simulink model "PMSM_ClosedLoop_s32k144"  (Simulink 9.0)
settings: Solver=FixedStepDiscrete  StartTime=0.0  StopTime=10  RelTol=1e-3  EnableMultiTasking=on
InitFcn:
  | mbd_s32k_consistency_checks(bdroot(gcs));
undefined symbols (not defined in the file): External, LQFP, One, Shot, TRGMUX_PDB_TRIG
libraries: mbd_s32k1xx_ec_toolbox x50, ammclib_bam_s32k14x x26, simulink x18, mbd_msd_ec_toolbox x5
(part 2 of 2)

== system PMSM_ClosedLoop_s32k144/S32K144 EVB/SlowLoopControl/Compute_Positioning_Mode ==
  Speed_Ref : Inport
  ABS : ammclib_bam_s32k14x/MLIB/bam_flt/MLIB_Abs_FLT
  Data Store Write : DataStoreWrite  DataStoreName=MODE
  Data Store Write2 : DataStoreWrite  DataStoreName=SPEED_REF
  Positioning_Mode : Stateflow chart  TreatAsAtomicUnit=on
      settings: RTWSystemCode=Nonreusable function  RTWFcnNameOpts=Use subsystem name  RTWFileNameOpts=Use subsystem name
  wires:
  Speed_Ref/1 -> ABS/1, Data Store Write2/1
  Positioning_Mode/1(Mode) -> Data Store Write/1
  ABS/1 -> Positioning_Mode/1(SPEED_REF)

== system PMSM_ClosedLoop_s32k144/S32K144 EVB/SlowLoopControl/Generate_Speed_Reference ==
  Speed_Cmd : Inport
  Align Sequence : Stateflow chart  TreatAsAtomicUnit=on
  AlignTimer : DataStoreMemory  DataStoreName=AlignTimer  ReadBeforeWriteMsg=warning  WriteAfterWriteMsg=warning  WriteAfterReadMsg=warning  ShowAdditionalParam=off  OutDataTypeStr=uint16
      settings: RTWStateStorageClass=ExportedGlobal
  AlignTimerIn : DataStoreRead  DataStoreName=AlignTimer
  AlignTimerOut : DataStoreWrite  DataStoreName=AlignTimer
  ExecureAlign : DataStoreWrite  DataStoreName=ExecuteAlign
  GFLIB_Ramp_FLT : ammclib_bam_s32k14x/GFLIB/bam_flt/GFLIB_Ramp_FLT  fltRampUp=0.1  fltRampDown=0.1
  Speed_Ref : Outport
  wires:
  Align Sequence/1(DelayTimeOut) -> AlignTimerOut/1
  AlignTimerIn/1 -> Align Sequence/1(DelayTimeIn)
  Align Sequence/3(ExecuteAlign) -> ExecureAlign/1
  Align Sequence/2(SpeedOut) -> GFLIB_Ramp_FLT/1
  GFLIB_Ramp_FLT/1 -> Speed_Ref/1
  Speed_Cmd/1 -> Align Sequence/2(SpeedIn)

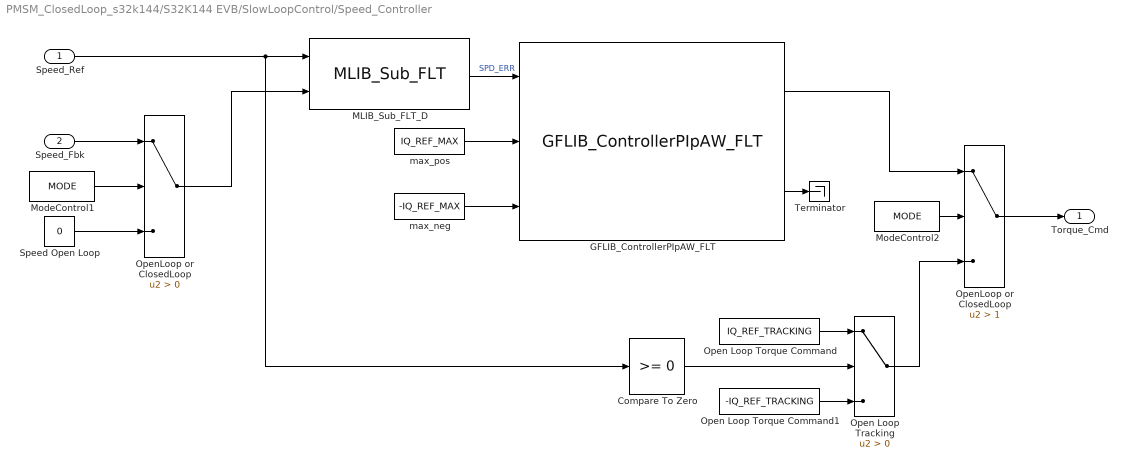
== system PMSM_ClosedLoop_s32k144/S32K144 EVB/SlowLoopControl/Speed_Controller ==
  Speed_Ref : Inport
  Speed_Fbk : Inport  Port=2
  Compare To Zero : simulink/Logic and Bit Operations/Compare To Zero  relop=>=  OutDataTypeStr=boolean
  GFLIB_ControllerPIpAW_FLT : ammclib_bam_s32k14x/GFLIB/bam_flt/GFLIB_ControllerPIpAW_FLT  fltPropGain=0.014207315561740161  fltIntegGain=0.00002231679909799742
  MLIB_Sub_FLT_D : ammclib_bam_s32k14x/MLIB/bam_flt/MLIB_Sub_FLT
  ModeControl1 : DataStoreRead  DataStoreName=MODE
  ModeControl2 : DataStoreRead  DataStoreName=MODE
  Open Loop Torque Command : Constant  Value=IQ_REF_TRACKING  OutDataTypeStr=Inherit: Inherit via back propagation
  Open Loop Torque Command1 : Constant  Value=-IQ_REF_TRACKING  OutDataTypeStr=Inherit: Inherit via back propagation
  Open Loop Tracking : Switch  Criteria=u2 > Threshold
  OpenLoop or ClosedLoop : Switch  Criteria=u2 > Threshold
  "OpenLoop or ClosedLoop " : Switch  Criteria=u2 > Threshold  Threshold=1
  Speed Open Loop : Constant  Value=0  OutDataTypeStr=Inherit: Inherit via back propagation
  Terminator : Terminator
  max_neg : Constant  Value=-IQ_REF_MAX  OutDataTypeStr=Inherit: Inherit via back propagation
  max_pos : Constant  Value=IQ_REF_MAX  OutDataTypeStr=Inherit: Inherit via back propagation
  Torque_Cmd : Outport
  wires:
  Speed_Ref/1 -> MLIB_Sub_FLT_D/1, Compare To Zero/1
  "OpenLoop or ClosedLoop "/1 -> Torque_Cmd/1
  Open Loop Tracking/1 -> "OpenLoop or ClosedLoop "/3
  Open Loop Torque Command/1 -> Open Loop Tracking/1
  Compare To Zero/1 -> Open Loop Tracking/2
  Open Loop Torque Command1/1 -> Open Loop Tracking/3
  GFLIB_ControllerPIpAW_FLT/1 -> "OpenLoop or ClosedLoop "/1
  ModeControl2/1 -> "OpenLoop or ClosedLoop "/2
  Speed Open Loop/1 -> OpenLoop or ClosedLoop/3
  ModeControl1/1 -> OpenLoop or ClosedLoop/2
  OpenLoop or ClosedLoop/1 -> MLIB_Sub_FLT_D/2
  Speed_Fbk/1 -> OpenLoop or ClosedLoop/1
  MLIB_Sub_FLT_D/1 -> GFLIB_ControllerPIpAW_FLT/1  "SPD_ERR"
  GFLIB_ControllerPIpAW_FLT/2 -> Terminator/1
  max_pos/1 -> GFLIB_ControllerPIpAW_FLT/2
  max_neg/1 -> GFLIB_ControllerPIpAW_FLT/3

== system PMSM_ClosedLoop_s32k144/S32K144 EVB/SlowLoopControl/Update_Theta_Offset ==
  Speed_Ref : Inport
  CW vs CCW : Switch  Criteria=u2 > Threshold
  Compare To Zero : simulink/Logic and Bit Operations/Compare To Zero  relop=>=  OutDataTypeStr=boolean
  Constant1 : Constant  Value=pi/2  OutDataTypeStr=Inherit: Inherit via back propagation
  Constant2 : Constant  Value=3*pi/2  OutDataTypeStr=Inherit: Inherit via back propagation
  Theta_Offset : DataStoreWrite  DataStoreName=THETA_OFFSET
  wires:
  Constant2/1 -> CW vs CCW/3
  CW vs CCW/1 -> Theta_Offset/1
  Compare To Zero/1 -> CW vs CCW/2
  Constant1/1 -> CW vs CCW/1
  Speed_Ref/1 -> Compare To Zero/1

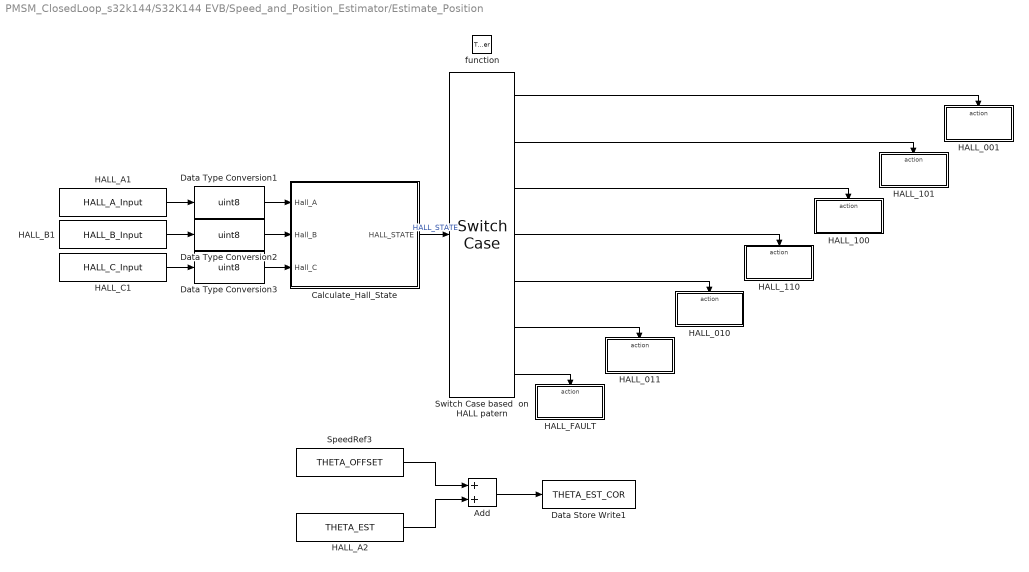
== system PMSM_ClosedLoop_s32k144/S32K144 EVB/Speed_and_Position_Estimator/Estimate_Position ==
  function : TriggerPort  TriggerType=function-call  VariantControl=(inherit)
  Add : Sum
  Calculate_Hall_State : Subsystem  Priority=1
  Data Store Write1 : DataStoreWrite  Priority=20  DataStoreName=THETA_EST_COR
  Data Type Conversion1 : DataTypeConversion  OutDataTypeStr=uint8
  Data Type Conversion2 : DataTypeConversion  OutDataTypeStr=uint8
  Data Type Conversion3 : DataTypeConversion  OutDataTypeStr=uint8
  HALL_001 : Subsystem  TreatAsAtomicUnit=on
  HALL_010 : Subsystem  TreatAsAtomicUnit=on
  HALL_011 : Subsystem  TreatAsAtomicUnit=on
  HALL_100 : Subsystem  TreatAsAtomicUnit=on
  HALL_101 : Subsystem  TreatAsAtomicUnit=on
  HALL_110 : Subsystem  TreatAsAtomicUnit=on
  HALL_A1 : DataStoreRead  DataStoreName=HALL_A_Input
  HALL_A2 : DataStoreRead  DataStoreName=THETA_EST
  HALL_B1 : DataStoreRead  DataStoreName=HALL_B_Input
  HALL_C1 : DataStoreRead  DataStoreName=HALL_C_Input
  HALL_FAULT : Subsystem  TreatAsAtomicUnit=on
  SpeedRef3 : DataStoreRead  DataStoreName=THETA_OFFSET
  Switch Case based  on HALL patern : SwitchCase  Priority=2  CaseConditions={1, 5, 4, 6, 2, 3}
  wires:
  Data Type Conversion2/1 -> Calculate_Hall_State/2(Hall_B)
  HALL_A1/1 -> Data Type Conversion1/1
  HALL_C1/1 -> Data Type Conversion3/1
  Data Type Conversion3/1 -> Calculate_Hall_State/3(Hall_C)
  Data Type Conversion1/1 -> Calculate_Hall_State/1(Hall_A)
  HALL_B1/1 -> Data Type Conversion2/1
  Calculate_Hall_State/1(HALL_STATE) -> Switch Case based  on HALL patern/1  "HALL_STATE"
  Switch Case based  on HALL patern/1 -> HALL_001/Action
  Switch Case based  on HALL patern/2 -> HALL_101/Action
  Switch Case based  on HALL patern/3 -> HALL_100/Action
  Switch Case based  on HALL patern/4 -> HALL_110/Action
  Switch Case based  on HALL patern/5 -> HALL_010/Action
  Switch Case based  on HALL patern/6 -> HALL_011/Action
  SpeedRef3/1 -> Add/1
  HALL_A2/1 -> Add/2
  Add/1 -> Data Store Write1/1
  Switch Case based  on HALL patern/7 -> HALL_FAULT/Action

== system PMSM_ClosedLoop_s32k144/S32K144 EVB/Speed_and_Position_Estimator/Update_HALL_A ==
  function : TriggerPort  TriggerType=function-call  VariantControl=(inherit)
  Data Store Read1 : DataStoreRead  DataStoreName=HALL_A_Input
  Data Store Write1 : DataStoreWrite  DataStoreName=HALL_A_Input
  Function-Call Generator : simulink/Ports & Subsystems/Function-Call Generator  sample_time=-1  numberOfIterations=1
  Logical Operator : Logic  Operator=NOT  AllPortsSameDT=off  OutDataTypeStr=boolean
  Call : Outport
  wires:
  Function-Call Generator/1 -> Call/1
  Data Store Read1/1 -> Logical Operator/1
  Logical Operator/1 -> Data Store Write1/1

== system PMSM_ClosedLoop_s32k144/S32K144 EVB/Speed_and_Position_Estimator/Update_HALL_B ==
  function : TriggerPort  TriggerType=function-call  VariantControl=(inherit)
  Data Store Read1 : DataStoreRead  DataStoreName=HALL_B_Input
  Data Store Write1 : DataStoreWrite  DataStoreName=HALL_B_Input
  Function-Call Generator : simulink/Ports & Subsystems/Function-Call Generator  sample_time=-1  numberOfIterations=1
  Logical Operator : Logic  Operator=NOT  AllPortsSameDT=off  OutDataTypeStr=boolean
  Call : Outport
  wires:
  Logical Operator/1 -> Data Store Write1/1
  Data Store Read1/1 -> Logical Operator/1
  Function-Call Generator/1 -> Call/1

== system PMSM_ClosedLoop_s32k144/S32K144 EVB/Speed_and_Position_Estimator/Update_HALL_C_Estimate_Speed ==
  function : TriggerPort  TriggerType=function-call  VariantControl=(inherit)
  Compute_Estimated_Speed : Subsystem  TreatAsAtomicUnit=on
  Data Store Read1 : DataStoreRead  Priority=0  DataStoreName=HALL_C_Input
  Data Store Write1 : DataStoreWrite  DataStoreName=HALL_C_Input
  Function-Call Generator : simulink/Ports & Subsystems/Function-Call Generator  sample_time=-1  numberOfIterations=1
  If : If  Priority=1  IfExpression=u1 == 1  ShowElse=off
  Logical Operator : Logic  Priority=2  Operator=NOT  AllPortsSameDT=off  OutDataTypeStr=boolean
  Call : Outport
  Speed_Fbk : Outport  Port=2
  wires:
  Function-Call Generator/1 -> Call/1
  Data Store Read1/1 -> If/1, Logical Operator/1
  Logical Operator/1 -> Data Store Write1/1
  If/1 -> Compute_Estimated_Speed/Action
  Compute_Estimated_Speed/1(Speed_Fbk) -> Speed_Fbk/1

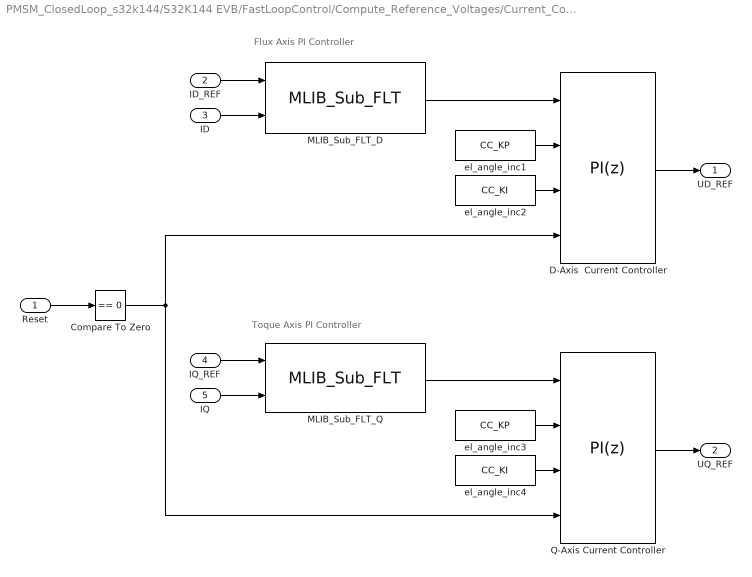
== system PMSM_ClosedLoop_s32k144/S32K144 EVB/FastLoopControl/Compute_Reference_Voltages/Current_Controllers_DQ ==
  note: Flux Axis PI Controller
  note: Toque Axis PI Controller
  Reset : Inport
  ID_REF : Inport  Port=2
  ID : Inport  Port=3
  IQ_REF : Inport  Port=4
  IQ : Inport  Port=5
  " D-Axis  Current Controller" : simulink/Continuous/PID Controller  Controller=PI  Form=Parallel  TimeDomain=Discrete-time  SampleTime=-1  IntegratorMethod=Forward Euler  FilterMethod=Forward Euler  ControllerParametersSource=external  P=1  I=1  D=0  UseFilter=on  N=100  TunerSelectOption=Transfer Function Based (PID Tuner App)  ZeroCross=off  InitialConditionSource=internal  InitialConditionForIntegrator=0  InitialConditionForFilter=0  DifferentiatorICPrevScaledInput=0  ExternalReset=rising  TrackingMode=off  Kt=1  LimitOutput=on  UpperSaturationLimit=0.9  LowerSaturationLimit=-0.9  LinearizeAsGain=off  AntiWindupMode=none  Kb=1  RndMeth=Simplest  POutMin=[]  POutMax=[]  IOutMin=[]  IOutMax=[]  DOutMin=[]  DOutMax=[]  NOutMin=[]  NOutMax=[]  SumOutMin=[]  SumOutMax=[]  SaturationOutMin=[]  SaturationOutMax=[]  PParamMin=[]  PParamMax=[]  IParamMin=[]  IParamMax=[]  DParamMin=[]  DParamMax=[]  NParamMin=[]  NParamMax=[]  KbParamMin=[]  KbParamMax=[]  KtParamMin=[]  KtParamMax=[]  KbOutMin=[]  KbOutMax=[]  KtOutMin=[]  KtOutMax=[]  IntegratorOutMin=[]  IntegratorOutMax=[]  FilterOutMin=[]  FilterOutMax=[]  SumI1OutMin=[]  SumI1OutMax=[]  SumI2OutMin=[]  SumI2OutMax=[]  SumI3OutMin=[]  SumI3OutMax=[]  SumDOutMin=[]  SumDOutMax=[]  DifferentiatorOutMin=[]  DifferentiatorOutMax=[]  FilterDiffOutCoefMin=[]  FilterDiffOutCoefMax=[]  ReciprocalOutMin=[]  ReciprocalOutMax=[]  SumDenOutMin=[]  SumDenOutMax=[]  SumNumOutMin=[]  SumNumOutMax=[]  DivideOutMin=[]  DivideOutMax=[]  IntegratorContinuousStateAttributes=''  IntegratorStateMustResolveToSignalObject=off  IntegratorRTWStateStorageClass=Auto  FilterContinuousStateAttributes=''  FilterStateMustResolveToSignalObject=off  FilterRTWStateStorageClass=Auto
  Compare To Zero : simulink/Logic and Bit Operations/Compare To Zero  relop===  OutDataTypeStr=boolean
  MLIB_Sub_FLT_D : ammclib_bam_s32k14x/MLIB/bam_flt/MLIB_Sub_FLT
  MLIB_Sub_FLT_Q : ammclib_bam_s32k14x/MLIB/bam_flt/MLIB_Sub_FLT
  Q-Axis Current Controller : simulink/Continuous/PID Controller  Controller=PI  Form=Parallel  TimeDomain=Discrete-time  SampleTime=-1  IntegratorMethod=Forward Euler  FilterMethod=Forward Euler  ControllerParametersSource=external  P=1  I=1  D=0  UseFilter=on  N=100  TunerSelectOption=Transfer Function Based (PID Tuner App)  ZeroCross=off  InitialConditionSource=internal  InitialConditionForIntegrator=0  InitialConditionForFilter=0  DifferentiatorICPrevScaledInput=0  ExternalReset=rising  TrackingMode=off  Kt=1  LimitOutput=on  UpperSaturationLimit=0.9  LowerSaturationLimit=-0.9  LinearizeAsGain=off  AntiWindupMode=clamping  Kb=1  RndMeth=Simplest  POutMin=[]  POutMax=[]  IOutMin=[]  IOutMax=[]  DOutMin=[]  DOutMax=[]  NOutMin=[]  NOutMax=[]  SumOutMin=[]  SumOutMax=[]  SaturationOutMin=[]  SaturationOutMax=[]  PParamMin=[]  PParamMax=[]  IParamMin=[]  IParamMax=[]  DParamMin=[]  DParamMax=[]  NParamMin=[]  NParamMax=[]  KbParamMin=[]  KbParamMax=[]  KtParamMin=[]  KtParamMax=[]  KbOutMin=[]  KbOutMax=[]  KtOutMin=[]  KtOutMax=[]  IntegratorOutMin=[]  IntegratorOutMax=[]  FilterOutMin=[]  FilterOutMax=[]  SumI1OutMin=[]  SumI1OutMax=[]  SumI2OutMin=[]  SumI2OutMax=[]  SumI3OutMin=[]  SumI3OutMax=[]  SumDOutMin=[]  SumDOutMax=[]  DifferentiatorOutMin=[]  DifferentiatorOutMax=[]  FilterDiffOutCoefMin=[]  FilterDiffOutCoefMax=[]  ReciprocalOutMin=[]  ReciprocalOutMax=[]  SumDenOutMin=[]  SumDenOutMax=[]  SumNumOutMin=[]  SumNumOutMax=[]  DivideOutMin=[]  DivideOutMax=[]  IntegratorContinuousStateAttributes=''  IntegratorStateMustResolveToSignalObject=off  IntegratorRTWStateStorageClass=Auto  FilterContinuousStateAttributes=''  FilterStateMustResolveToSignalObject=off  FilterRTWStateStorageClass=Auto
  el_angle_inc1 : DataStoreRead  DataStoreName=CC_KP
  el_angle_inc2 : DataStoreRead  DataStoreName=CC_KI
  el_angle_inc3 : DataStoreRead  DataStoreName=CC_KP
  el_angle_inc4 : DataStoreRead  DataStoreName=CC_KI
  UD_REF : Outport
  UQ_REF : Outport  Port=2
  wires:
  MLIB_Sub_FLT_D/1 -> " D-Axis  Current Controller"/1
  el_angle_inc1/1 -> " D-Axis  Current Controller"/2
  el_angle_inc2/1 -> " D-Axis  Current Controller"/3
  ID_REF/1 -> MLIB_Sub_FLT_D/1
  MLIB_Sub_FLT_Q/1 -> Q-Axis Current Controller/1
  el_angle_inc3/1 -> Q-Axis Current Controller/2
  el_angle_inc4/1 -> Q-Axis Current Controller/3
  ID/1 -> MLIB_Sub_FLT_D/2
  IQ_REF/1 -> MLIB_Sub_FLT_Q/1
  IQ/1 -> MLIB_Sub_FLT_Q/2
  " D-Axis  Current Controller"/1 -> UD_REF/1
  Q-Axis Current Controller/1 -> UQ_REF/1
  Reset/1 -> Compare To Zero/1
  Compare To Zero/1 -> Q-Axis Current Controller/4, " D-Axis  Current Controller"/4

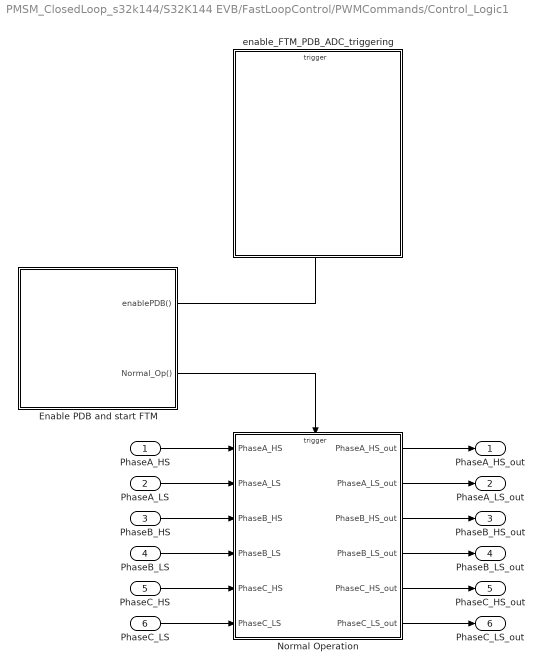
== system PMSM_ClosedLoop_s32k144/S32K144 EVB/FastLoopControl/PWMCommands/Control_Logic1 ==
  PhaseA_HS : Inport
  PhaseA_LS : Inport  Port=2
  PhaseB_HS : Inport  Port=3
  PhaseB_LS : Inport  Port=4
  PhaseC_HS : Inport  Port=5
  PhaseC_LS : Inport  Port=6
  Enable PDB and start FTM : Stateflow chart  TreatAsAtomicUnit=on
  Normal Operation : Subsystem  TreatAsAtomicUnit=on
  enable_FTM_PDB_ADC_triggering : Subsystem  TreatAsAtomicUnit=on
      settings: RTWSystemCode=Inline
  PhaseA_HS_out : Outport
  PhaseA_LS_out : Outport  Port=2
  PhaseB_HS_out : Outport  Port=3
  PhaseB_LS_out : Outport  Port=4
  PhaseC_HS_out : Outport  Port=5
  PhaseC_LS_out : Outport  Port=6
  wires:
  Enable PDB and start FTM/2(Normal_Op()) -> Normal Operation/Trigger
  Enable PDB and start FTM/1(enablePDB()) -> enable_FTM_PDB_ADC_triggering/Trigger
  PhaseB_HS/1 -> Normal Operation/3(PhaseB_HS)
  PhaseB_LS/1 -> Normal Operation/4(PhaseB_LS)
  PhaseA_LS/1 -> Normal Operation/2(PhaseA_LS)
  PhaseC_HS/1 -> Normal Operation/5(PhaseC_HS)
  PhaseA_HS/1 -> Normal Operation/1(PhaseA_HS)
  PhaseC_LS/1 -> Normal Operation/6(PhaseC_LS)
  Normal Operation/6(PhaseC_LS_out) -> PhaseC_LS_out/1
  Normal Operation/5(PhaseC_HS_out) -> PhaseC_HS_out/1
  Normal Operation/4(PhaseB_LS_out) -> PhaseB_LS_out/1
  Normal Operation/3(PhaseB_HS_out) -> PhaseB_HS_out/1
  Normal Operation/2(PhaseA_LS_out) -> PhaseA_LS_out/1
  Normal Operation/1(PhaseA_HS_out) -> PhaseA_HS_out/1

== system PMSM_ClosedLoop_s32k144/S32K144 EVB/FastLoopControl/Rotor_Position/ComputeElectricAngle ==
  Speed_Reference [rad/s] : Inport
  DIV : ammclib_bam_s32k14x/MLIB/bam_flt/MLIB_Div_FLT
  GFLIB_IntegratorTR_F32 : ammclib_bam_s32k14x/GFLIB/bam_f32/GFLIB_IntegratorTR_F32  f32C1=(2*pi/60)*PP*Nmax*(C_LST/2/pi)*(2^31)  u16NShift=0
  MLIB_ConvertPU_F32FLT : ammclib_bam_s32k14x/MLIB/bam_f32/MLIB_ConvertPU_F32FLT
  MLIB_ConvertPU_FLTF32 : ammclib_bam_s32k14x/MLIB/bam_flt/MLIB_ConvertPU_FLTF32
  MUL : ammclib_bam_s32k14x/MLIB/bam_flt/MLIB_Mul_FLT
  SpeedMax_rad/s : Constant  Value=Nmax*(2*pi/60)  OutDataTypeStr=Inherit: Inherit via back propagation
  pi : Constant  Value=pi  OutDataTypeStr=Inherit: Inherit via back propagation
  theta : Outport  OutDataTypeStr=single
  wires:
  pi/1 -> MUL/2
  GFLIB_IntegratorTR_F32/1 -> MLIB_ConvertPU_FLTF32/1
  MLIB_ConvertPU_F32FLT/1 -> GFLIB_IntegratorTR_F32/1
  MLIB_ConvertPU_FLTF32/1 -> MUL/1
  MUL/1 -> theta/1
  Speed_Reference [rad/s]/1 -> DIV/1
  DIV/1 -> MLIB_ConvertPU_F32FLT/1
  SpeedMax_rad/s/1 -> DIV/2

== system PMSM_ClosedLoop_s32k144/S32K144 EVB/IO Controls/NormalOp/FAULT ==
  Action Port : ActionPort
  LED_BLUE : mbd_s32k1xx_ec_toolbox/GPIO Blocks/Digital_Output  gpio_pin=PTD0: [PTD0 | Port D I/O]  init_val=Low  drive_strength=Low
  LED_RED : mbd_s32k1xx_ec_toolbox/GPIO Blocks/Digital_Output  gpio_pin=PTD15: [PTD15 | Port D I/O]  init_val=Low  drive_strength=Low
  OFF : Constant  OutDataTypeStr=boolean
  ON : Constant  Value=0  OutDataTypeStr=boolean
  wires:
  OFF/1 -> LED_BLUE/1
  ON/1 -> LED_RED/1

== system PMSM_ClosedLoop_s32k144/S32K144 EVB/IO Controls/NormalOp/RUNNING_OK ==
  Action Port : ActionPort
  LED_BLUE : mbd_s32k1xx_ec_toolbox/GPIO Blocks/Digital_Output  gpio_pin=PTD0: [PTD0 | Port D I/O]  init_val=Low  drive_strength=Low
  LED_RED : mbd_s32k1xx_ec_toolbox/GPIO Blocks/Digital_Output  gpio_pin=PTD15: [PTD15 | Port D I/O]  init_val=Low  drive_strength=Low
  OFF : Constant  OutDataTypeStr=boolean
  ON : Constant  Value=0  OutDataTypeStr=boolean
  wires:
  OFF/1 -> LED_RED/1
  ON/1 -> LED_BLUE/1

== system PMSM_ClosedLoop_s32k144/S32K144 EVB/IO Controls/WaitForStart/Check_Hall_Error ==
  H1 : Inport
  H2 : Inport  Port=2
  H3 : Inport  Port=3
  Add : Sum  Inputs=+++
  Compare To Constant : simulink/Logic and Bit Operations/Compare To Constant  relop===  const=3  OutDataTypeStr=boolean
  Compare To Constant1 : simulink/Logic and Bit Operations/Compare To Constant  relop===  const=0  OutDataTypeStr=boolean
  Logical Operator : Logic  Operator=OR  AllPortsSameDT=off  OutDataTypeStr=boolean
  Hall_Errorr : Outport
  wires:
  Logical Operator/1 -> Hall_Errorr/1
  Compare To Constant1/1 -> Logical Operator/2
  H3/1 -> Add/3
  Add/1 -> Compare To Constant1/1, Compare To Constant/1
  H2/1 -> Add/2
  Compare To Constant/1 -> Logical Operator/1
  H1/1 -> Add/1

== system PMSM_ClosedLoop_s32k144/S32K144 EVB/IO Controls/WaitForStart/HALL_FAULT ==
  Action Port : ActionPort
  Data Store Write2 : DataStoreWrite  DataStoreName=HALL_ERROR
  "NOK " : Constant  OutDataTypeStr=uint8
  wires:
  "NOK "/1 -> Data Store Write2/1

== system PMSM_ClosedLoop_s32k144/S32K144 EVB/IRQ_Dispatcher/Generate_Triggers/Keep_Counting ==
  LoopCounter : Inport
  Action Port : ActionPort
  LoopCounter_save : DataStoreWrite  DataStoreName=LoopCounter
  wires:
  LoopCounter/1 -> LoopCounter_save/1

== system PMSM_ClosedLoop_s32k144/S32K144 EVB/IRQ_Dispatcher/Generate_Triggers/Trigger_SlowLoop_Execution ==
  Action Port : ActionPort
  Function-Call Generator : simulink/Ports & Subsystems/Function-Call Generator  sample_time=-1  numberOfIterations=1
  LoopCounter_reset : DataStoreWrite  DataStoreName=LoopCounter
  reset_to_zero : Constant  Value=0  OutDataTypeStr=uint16
  Call : Outport
  wires:
  Function-Call Generator/1 -> Call/1
  reset_to_zero/1 -> LoopCounter_reset/1

== system PMSM_ClosedLoop_s32k144/S32K144 EVB/Measurements/FaultDetection/FAILURE ==
  Action Port : ActionPort
  Compare To Two : simulink/Logic and Bit Operations/Compare To Constant  relop=>=  const=2  OutDataTypeStr=boolean
  FAULT_read : DataStoreRead  DataStoreName=FAULT
  Failed Subsystem : Subsystem  TreatAsAtomicUnit=on
  If : If  NumInputs=2  IfExpression=(u1 == 1)&(u2==1)  ShowElse=off
  LoopCounter_read : DataStoreRead  DataStoreName=LoopCounter
  wires:
  If/1 -> Failed Subsystem/Action
  LoopCounter_read/1 -> Compare To Two/1
  FAULT_read/1 -> If/1
  Compare To Two/1 -> If/2

== system PMSM_ClosedLoop_s32k144/S32K144 EVB/Speed_and_Position_Estimator/Estimate_Position/Calculate_Hall_State ==
  Hall_A : Inport
  Hall_B : Inport  Port=2
  Hall_C : Inport  Port=3
  Gain1 : Gain  Gain=4  OutDataTypeStr=uint8  ParamDataTypeStr=Inherit: Same as input
  Gain2 : Gain  Gain=2  OutDataTypeStr=uint8  ParamDataTypeStr=Inherit: Same as input
  Sum : Sum  Inputs=+++  AccumDataTypeStr=uint8  OutDataTypeStr=uint8  InputSameDT=on
  HALL_STATE : Outport
  wires:
  Sum/1 -> HALL_STATE/1
  Gain2/1 -> Sum/2
  Gain1/1 -> Sum/1
  Hall_A/1 -> Gain1/1
  Hall_B/1 -> Gain2/1
  Hall_C/1 -> Sum/3

== system PMSM_ClosedLoop_s32k144/S32K144 EVB/Speed_and_Position_Estimator/Estimate_Position/HALL_001 ==
  Action Port : ActionPort
  -180deg : Constant  Value=-pi  OutDataTypeStr=Inherit: Inherit via back propagation
  Data Store Write4 : DataStoreWrite  DataStoreName=THETA_EST
  wires:
  -180deg/1 -> Data Store Write4/1

== system PMSM_ClosedLoop_s32k144/S32K144 EVB/Speed_and_Position_Estimator/Estimate_Position/HALL_010 ==
  Action Port : ActionPort
  60deg : Constant  Value=pi/3  OutDataTypeStr=Inherit: Inherit via back propagation
  Data Store Write4 : DataStoreWrite  DataStoreName=THETA_EST
  wires:
  60deg/1 -> Data Store Write4/1

== system PMSM_ClosedLoop_s32k144/S32K144 EVB/Speed_and_Position_Estimator/Estimate_Position/HALL_011 ==
  Action Port : ActionPort
  120deg : Constant  Value=2*pi/3  OutDataTypeStr=Inherit: Inherit via back propagation
  Data Store Write4 : DataStoreWrite  DataStoreName=THETA_EST
  wires:
  120deg/1 -> Data Store Write4/1

== system PMSM_ClosedLoop_s32k144/S32K144 EVB/Speed_and_Position_Estimator/Estimate_Position/HALL_100 ==
  Action Port : ActionPort
  -60deg : Constant  Value=-pi/3  OutDataTypeStr=Inherit: Inherit via back propagation
  Data Store Write4 : DataStoreWrite  DataStoreName=THETA_EST
  wires:
  -60deg/1 -> Data Store Write4/1

== system PMSM_ClosedLoop_s32k144/S32K144 EVB/Speed_and_Position_Estimator/Estimate_Position/HALL_101 ==
  Action Port : ActionPort
  -120deg : Constant  Value=-2*pi/3  OutDataTypeStr=Inherit: Inherit via back propagation
  Data Store Write4 : DataStoreWrite  DataStoreName=THETA_EST
  wires:
  -120deg/1 -> Data Store Write4/1

== system PMSM_ClosedLoop_s32k144/S32K144 EVB/Speed_and_Position_Estimator/Estimate_Position/HALL_110 ==
  Action Port : ActionPort
  0deg : Constant  Value=0  OutDataTypeStr=Inherit: Inherit via back propagation
  Data Store Write4 : DataStoreWrite  DataStoreName=THETA_EST
  wires:
  0deg/1 -> Data Store Write4/1

== system PMSM_ClosedLoop_s32k144/S32K144 EVB/Speed_and_Position_Estimator/Estimate_Position/HALL_FAULT ==
  Action Port : ActionPort
  Data Store Write1 : DataStoreWrite  DataStoreName=FAULT
  Data Store Write2 : DataStoreWrite  DataStoreName=HALL_ERROR
  FTM_PWM_Disable_Enable : mbd_s32k1xx_ec_toolbox/Motor Control Blocks/FTM Blocks/FTM_PWM_Disable_Enable  ftmModule=3  action=Disable
  NOK : Constant  OutDataTypeStr=boolean
  "NOK " : Constant  OutDataTypeStr=uint8
  wires:
  NOK/1 -> Data Store Write1/1
  "NOK "/1 -> Data Store Write2/1

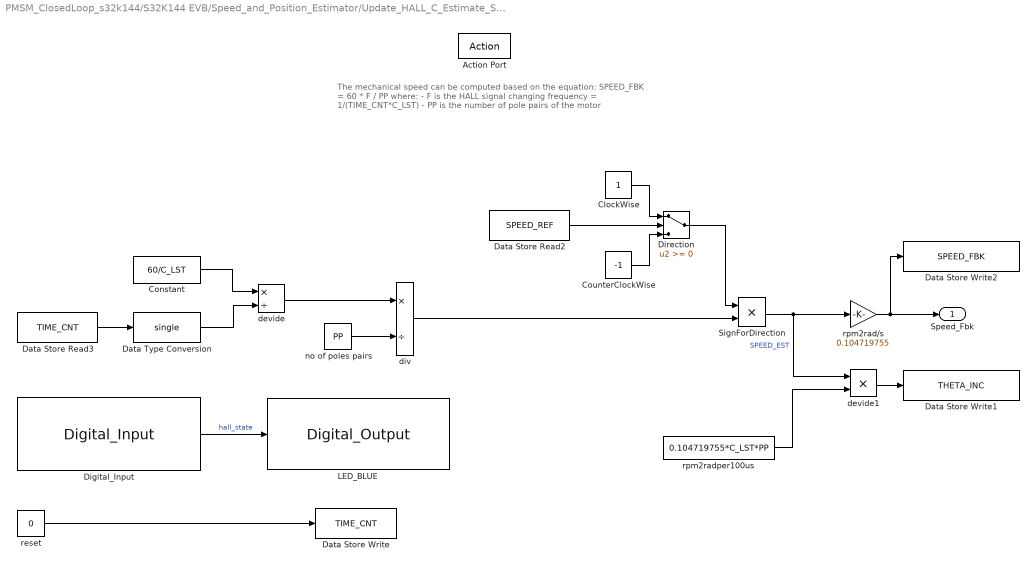
== system PMSM_ClosedLoop_s32k144/S32K144 EVB/Speed_and_Position_Estimator/Update_HALL_C_Estimate_Speed/Compute_Estimated_Speed ==
  note: The mechanical speed can be computed based on the equation:
      | SPEED_FBK = 60 * F / PP
      | where:
      | - F is the HALL signal changing frequency = 1/(TIME_CNT*C_LST)
      | - PP is the number of pole pairs of the motor
  Action Port : ActionPort
  ClockWise : Constant  OutDataTypeStr=Inherit: Inherit via back propagation
  Constant : Constant  Value=60/C_LST  OutDataTypeStr=single
  CounterClockWise : Constant  Value=-1  OutDataTypeStr=Inherit: Inherit via back propagation
  Data Store Read2 : DataStoreRead  DataStoreName=SPEED_REF
  Data Store Read3 : DataStoreRead  DataStoreName=TIME_CNT
  Data Store Write : DataStoreWrite  DataStoreName=TIME_CNT
  Data Store Write1 : DataStoreWrite  Priority=1  DataStoreName=THETA_INC
  Data Store Write2 : DataStoreWrite  Priority=1  DataStoreName=SPEED_FBK
  Data Type Conversion : DataTypeConversion  OutDataTypeStr=single
  Digital_Input : mbd_s32k1xx_ec_toolbox/GPIO Blocks/Digital_Input  gpio_pin=PTA1: [PTA1 | Port A I/O]  pull_resistor=None  passive_filter=off
  Direction : Switch  OutDataTypeStr=single
  LED_BLUE : mbd_s32k1xx_ec_toolbox/GPIO Blocks/Digital_Output  gpio_pin=PTD0: [PTD0 | Port D I/O]  init_val=Low  drive_strength=Low
  SignForDirection : Product  Inputs=**  OutDataTypeStr=single  RndMeth=Zero
  devide : Product  Inputs=*/  OutDataTypeStr=single
  devide1 : Product  Inputs=**  OutDataTypeStr=single
  div : Product  Priority=0  Inputs=*/  OutDataTypeStr=single
  no of poles pairs : Constant  Value=PP  OutDataTypeStr=single
  reset : Constant  Value=0  OutDataTypeStr=uint32
  rpm2rad/s : Gain  Gain=0.104719755
  rpm2radper100us : Constant  Value=0.104719755*C_LST*PP  OutDataTypeStr=single
  Speed_Fbk : Outport
  wires:
  Data Store Read3/1 -> Data Type Conversion/1
  Data Type Conversion/1 -> devide/2
  Constant/1 -> devide/1
  devide/1 -> div/1
  no of poles pairs/1 -> div/2
  Data Store Read2/1 -> Direction/2
  ClockWise/1 -> Direction/1
  CounterClockWise/1 -> Direction/3
  Direction/1 -> SignForDirection/1
  SignForDirection/1 -> rpm2rad/s/1, devide1/1  "SPEED_EST"
  div/1 -> SignForDirection/2
  reset/1 -> Data Store Write/1
  rpm2radper100us/1 -> devide1/2
  devide1/1 -> Data Store Write1/1
  Digital_Input/1 -> LED_BLUE/1  "hall_state"
  rpm2rad/s/1 -> Data Store Write2/1, Speed_Fbk/1

== system PMSM_ClosedLoop_s32k144/S32K144 EVB/FastLoopControl/PWMCommands/Control_Logic1/Normal Operation ==
  PhaseA_HS : Inport
  PhaseA_LS : Inport  Port=2
  PhaseB_HS : Inport  Port=3
  PhaseB_LS : Inport  Port=4
  PhaseC_HS : Inport  Port=5
  PhaseC_LS : Inport  Port=6
  function : TriggerPort  TriggerType=function-call  VariantControl=(inherit)
  PhaseA_HS_out : Outport
  PhaseA_LS_out : Outport  Port=2
  PhaseB_HS_out : Outport  Port=3
  PhaseB_LS_out : Outport  Port=4
  PhaseC_HS_out : Outport  Port=5
  PhaseC_LS_out : Outport  Port=6
  wires:
  PhaseA_HS/1 -> PhaseA_HS_out/1
  PhaseA_LS/1 -> PhaseA_LS_out/1
  PhaseB_HS/1 -> PhaseB_HS_out/1
  PhaseB_LS/1 -> PhaseB_LS_out/1
  PhaseC_HS/1 -> PhaseC_HS_out/1
  PhaseC_LS/1 -> PhaseC_LS_out/1

== system PMSM_ClosedLoop_s32k144/S32K144 EVB/FastLoopControl/PWMCommands/Control_Logic1/enable_FTM_PDB_ADC_triggering ==
  function : TriggerPort  TriggerType=function-call  VariantControl=(inherit)
  Custom code to reload the PDB value : Subsystem  Priority=6  mask(System Outputs){ShowInLibBrowser=0}
      mask prompts: ShowInLibBrowser "Simulink:masks:CustCodeMaskParam1_MP"
      settings: CopyFcn=cccopyfcn(gcb)  OpenFcn=ccopenfcn('System Outputs Function')
      mask Help: eval('feval(''rtwprivate'',''rtwhelpview'',''rtw_sys_outputs_block'')');
      mask Display: disp('System\nOutputs');
  FTM_Init_Trigger_Disable_Enable : mbd_s32k1xx_ec_toolbox/Motor Control Blocks/FTM Blocks/FTM_Init_Trigger_Disable_Enable  Priority=3  ftmModule=3  action=Enable
  FTM_PWM_Disable_Enable : mbd_s32k1xx_ec_toolbox/Motor Control Blocks/FTM Blocks/FTM_PWM_Disable_Enable  Priority=1  ftmModule=3  action=Enable
  ON : Constant  Priority=2  OutDataTypeStr=boolean
  PDB0_Enable : mbd_s32k1xx_ec_toolbox/Motor Control Blocks/PDB Blocks/PDB_Enable  Priority=4  pdbModule=0  pdbAction=Enable
  PDB1_Enable : mbd_s32k1xx_ec_toolbox/Motor Control Blocks/PDB Blocks/PDB_Enable  Priority=5  pdbModule=1  pdbAction=Enable
  "SpeedCmd " : DataStoreWrite  DataStoreName=READY
  TPP_ISR_Enable_Disable 1 : mbd_msd_ec_toolbox/TPP/TPP_ISR_Enable_Disable  Priority=7  tppInstance=0  mcuTppIntEn=on  prioInt=15
  wires:
  ON/1 -> "SpeedCmd "/1

== system PMSM_ClosedLoop_s32k144/S32K144 EVB/Measurements/FaultDetection/FAILURE/Failed Subsystem ==
  Action Port : ActionPort
  FAULT_write : DataStoreWrite  DataStoreName=FAULT
  FTM_PWM_Disable_Enable : mbd_s32k1xx_ec_toolbox/Motor Control Blocks/FTM Blocks/FTM_PWM_Disable_Enable  Priority=1  ftmModule=3  action=Disable
  NOK : Constant  OutDataTypeStr=boolean
  TPP_Functional_Mode : mbd_msd_ec_toolbox/TPP/TPP_Functional_Mode  tppInstance=0  action=Sleep
  wires:
  NOK/1 -> FAULT_write/1

== system PMSM_ClosedLoop_s32k144/S32K144 EVB/FastLoopControl/PWMCommands/Control_Logic1/enable_FTM_PDB_ADC_triggering/Custom code to reload the PDB value ==

== stateflow chart S32K144 EVB/SlowLoopControl/Generate_Speed_Reference/Align Sequence ==
  settings: sampleTime=0.500
  note: Delay for 3 seconds.
  (default) -> (junction 9)
  (junction 9) -> (junction 10) [order 1] : [DelayTimeIn > 3000]
      | {SpeedOut = SpeedIn;
      | ExecuteAlign = 0;}
  (junction 9) -> (junction 11) [order 2]
  (junction 10) -> (junction 12)
  (junction 11) -> (junction 12) : {SpeedOut = 0;
      | DelayTimeOut = DelayTimeIn + 1;
      | ExecuteAlign = 1;}
  data: DelayTimeOut output uint16; DelayTimeIn input uint16; SpeedOut output single; SpeedIn input single; ExecuteAlign output boolean

== stateflow chart S32K144 EVB/FastLoopControl/PWMCommands/Control_Logic1/Enable PDB and start FTM ==
  settings: sampleTime=0.500
  state END
  state A
  (default) -> A
  A -> END : /*Post initializations*/
      | {enablePDB;}
  END -> END : {Normal_Op;}
  events: enablePDB output FUNCTION_CALL_EVENT; Normal_Op output FUNCTION_CALL_EVENT

== stateflow chart S32K144 EVB/SlowLoopControl/Compute_Positioning_Mode/Positioning_Mode ==
  note: Force Mode = 0 when speed is below specified value
      | Tracking Mode = 1 when speed is between specified values
      | Sensor/Sensorless Mode = 2 when speed is above specified value
  (default) -> (junction 34)
  (junction 34) -> (junction 35) [order 1] : [SPEED_REF < FORCE_MODE_SPEED] /* rad/s */
      | {Mode = 0;}
  (junction 34) -> (junction 36) [order 2]
  (junction 35) -> (junction 37)
  (junction 36) -> (junction 37) [order 1] : [(SPEED_REF >= (FORCE_MODE_SPEED)) && (SPEED_REF < (TRACKING_MODE_SPEED))] /* rad/s */
      | {Mode = 1;}
  (junction 36) -> (junction 38) [order 2]
  (junction 37) -> (junction 39)
  (junction 38) -> (junction 39) : {Mode = 2;}
  data: SPEED_REF input double; Mode output uint16; FORCE_MODE_SPEED parameter double; TRACKING_MODE_SPEED parameter double
